simulink model "pv_dq_sim"  (R2014b)
settings: Solver=ode45  SolverMode=SingleTasking  StartTime=0.0  StopTime=2  MaxStep=0.0002  RelTol=0.0001
values from neighbouring files (symbols this model uses):
  C = full(C)    [ex3busPV.m]    (also in ex_get_started_here.m = 5e-07; pv_dq.m = 4.01652892562e-06)
  Kci = Kcp^2/(2*Linv)    [exSyncGenPVinv.m]    (also in pv_dq.m = 3.11562907794)
  Kcp = 10*4*pi*Linv    [exSyncGenPVinv.m]    (also in pv_dq.m = 0.0495867768595)
  Kpi = 0.1*Kpp^2/(Ebus/Vinv_rt)    [exSyncGenPVinv.m]    (also in pv_dq.m = 251.934662919)
  Kpp = 200*(Ebus/Vinv_rt)    [exSyncGenPVinv.m]    (also in pv_dq.m = 12.596733146)
  L = 0.5    [ex2busStability.m]    (also in ex_get_started_here.m = 0.05; pv_dq.m = 0.000394599032459)
  Pdc_op = 0.6*Pinv_rt    [exSyncGenPVinv.m]    (also in pv_dq.m = 1600000)
  Qstar = 0    [exSyncGenPVinv.m]    (also in pv_dq.m)
  ramp_duration = 1    [pv_dq.m]
  ramp_size = -0.1    [pv_dq.m]
  ramp_starts_at = 0.2    [pv_dq.m]
  Vdcset = (2^0.5)*Vinv_rt/duty_max    [exSyncGenPVinv.m]    (also in pv_dq.m = 19958.8053116)
  Vg = 22e3 / 3^0.5    (= 12701.7059222)    [pv_dq.m]
  Vinv_rt = mpc.bus(ssgen(synrp),VM).*baseV(ssgen(synrp))    [exSyncGenPVinv.m]    (also in pv_dq.m = 12701.7059222)
  ws = 2*pi*50    (= 314.159265359)    [ex14busSGandPV.m]    (also in ex2busStability.m; ex3busPV.m; ex7busLongLine.m; ex9busSG.m)
undefined symbols (not defined in the file or in its folder): magnitude
libraries: simulink x1
settings Model: Creator=COPEC  LastModifiedBy=Juri
settings OptimizationCC: BlockReduction=off  BooleanDataType=off
settings DebuggingCC: SaveWithParameterizedLinksMsg=none  UnderspecifiedInitializationDetection=Classic  MergeDetectMultiDrivingBlocksExec=none  SignalResolutionControl=TryResolveAllWithWarning  SolverPrmCheckMsg=none  FrameProcessingCompatibilityMsg=error
settings HardwareCC: TargetUnknown=on

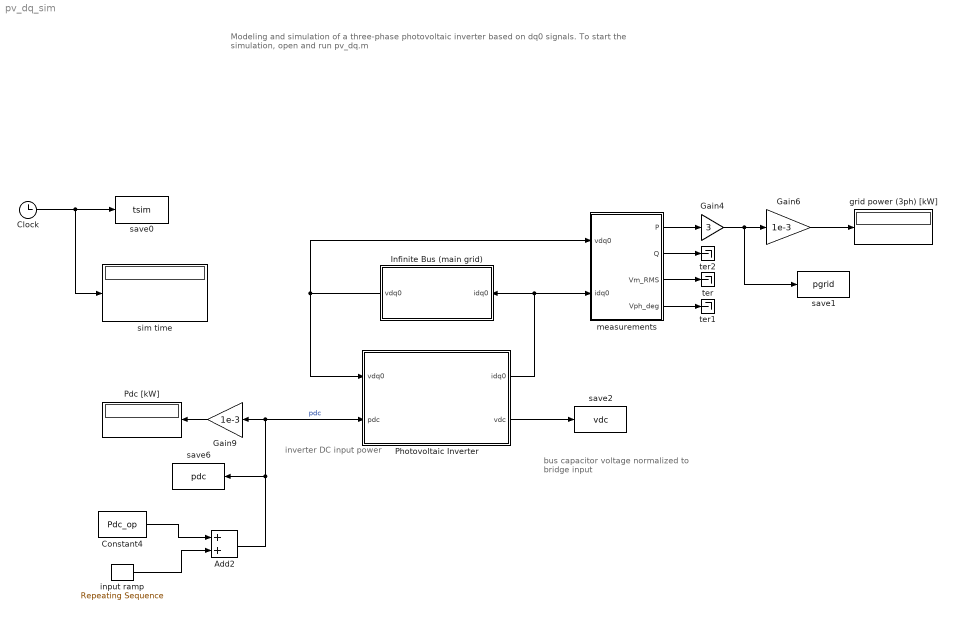
== system pv_dq_sim ==
  note: inverter DC input power
  note: bus capacitor voltage normalized to bridge input
  note: Modeling and simulation of a three-phase
      | photovoltaic inverter based on dq0 signals.
      |
      | To start the simulation, open and run pv_dq.m
  Add2 : Sum
  Clock : Clock
  Constant4 : Constant  Value=Pdc_op
  Gain4 : Gain  Gain=3
  Gain6 : Gain  Gain=1e-3
  Gain9 : Gain  Gain=1e-3
  Infinite Bus (main grid) : Subsystem
  Pdc [kW] : Display
  Photovoltaic Inverter : Subsystem
  grid power (3ph) [kW] : Display
  input ramp : simulink/Sources/Repeating Sequence  rep_seq_t=[0 ramp_starts_at (ramp_starts_at+ramp_duration) 1e6]  rep_seq_y=[0 0 Pdc_op*ramp_size Pdc_op*ramp_size]
  measurements : Subsystem
  save0 : ToWorkspace  VariableName=tsim  SampleTime=-1
  save1 : ToWorkspace  VariableName=pgrid  SampleTime=-1
  save2 : ToWorkspace  VariableName=vdc  SampleTime=-1
  save6 : ToWorkspace  VariableName=pdc  SampleTime=-1
  sim time : Display
  ter : Terminator
  ter1 : Terminator
  ter2 : Terminator
  wires:
  Clock/1 -> sim time/1, save0/1
  Gain6/1 -> grid power (3ph) [kW]/1
  input ramp/1 -> Add2/2
  Gain9/1 -> Pdc [kW]/1
  Constant4/1 -> Add2/1
  Add2/1 -> Photovoltaic Inverter/2(pdc), Gain9/1, save6/1  "pdc"
  Infinite Bus (main grid)/1(vdq0) -> measurements/1(vdq0), Photovoltaic Inverter/1(vdq0)
  Photovoltaic Inverter/1(idq0) -> Infinite Bus (main grid)/1(idq0), measurements/2(idq0)
  measurements/3(Vm_RMS) -> ter/1
  measurements/4(Vph_deg) -> ter1/1
  measurements/2(Q) -> ter2/1
  measurements/1(P) -> Gain4/1
  Gain4/1 -> Gain6/1, save1/1
  Photovoltaic Inverter/2(vdc) -> save2/1

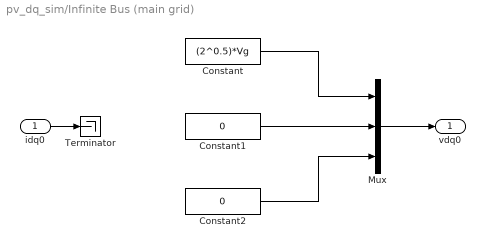
== system pv_dq_sim/Infinite Bus (main grid) ==
  idq0 : Inport
  Constant : Constant  Value=(2^0.5)*Vg
  Constant1 : Constant  Value=0
  Constant2 : Constant  Value=0
  Mux : Mux  Inputs=3
  Terminator : Terminator
  vdq0 : Outport
  wires:
  Mux/1 -> vdq0/1
  Constant/1 -> Mux/1
  Constant1/1 -> Mux/2
  Constant2/1 -> Mux/3
  idq0/1 -> Terminator/1

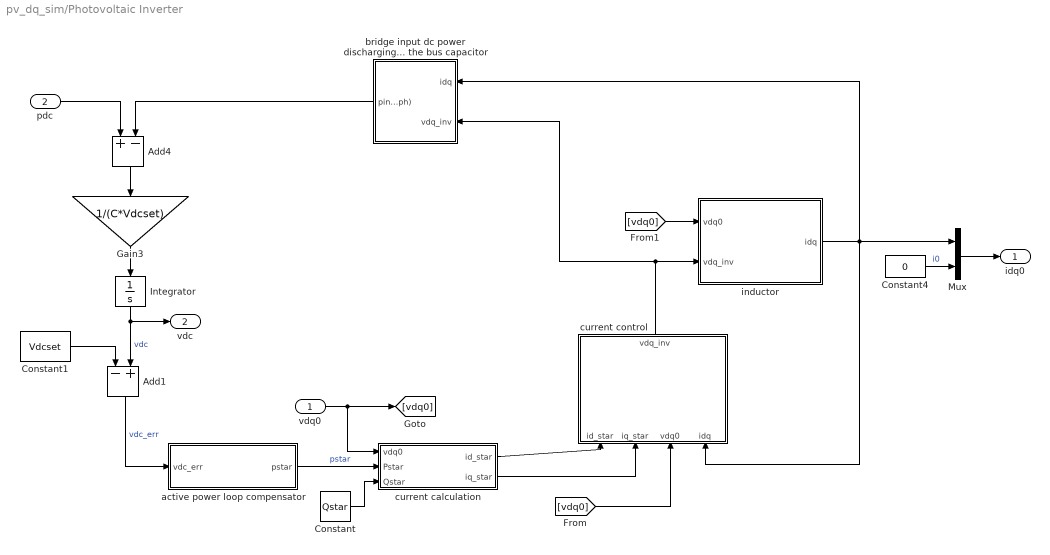
== system pv_dq_sim/Photovoltaic Inverter ==
  vdq0 : Inport
  pdc : Inport  Port=2
  Add1 : Sum  Inputs=-+
  Add4 : Sum  Inputs=+-
  Constant : Constant  Value=Qstar
  Constant1 : Constant  Value=Vdcset
  Constant4 : Constant  Value=0
  Gain3 : Gain  Gain=1/(C*Vdcset)
  Integrator : Integrator  InitialCondition=Vdcset
  Mux : Mux  Inputs=2
  active power loop compensator : Subsystem
  bridge input dc power discharging the bus capacitor : Subsystem
  current control : Subsystem
  current calculation : Subsystem
  inductor : Subsystem
  idq0 : Outport
  vdc : Outport  Port=2
  wires:
  Integrator/1 -> Add1/2, vdc/1  "vdc"
  Constant/1 -> current calculation/3(Qstar)
  Add4/1 -> Gain3/1
  Constant1/1 -> Add1/1
  active power loop compensator/1(pstar) -> current calculation/2(Pstar)  "pstar"
  Gain3/1 -> Integrator/1
  current calculation/2(iq_star) -> current control/2(iq_star)
  current calculation/1(id_star) -> current control/1(id_star)
  Add1/1 -> active power loop compensator/1(vdc_err)  "vdc_err"
  pdc/1 -> Add4/1
  vdq0/1 -> current calculation/1(vdq0), [vdq0]
  [vdq0] -> current control/3(vdq0)
  [vdq0] -> inductor/1(vdq0)
  current control/1(vdq_inv) -> bridge input dc power discharging the bus capacitor/2(vdq_inv), inductor/2(vdq_inv)
  bridge input dc power discharging the bus capacitor/1(pinv (3ph)) -> Add4/2
  Mux/1 -> idq0/1
  inductor/1(idq) -> bridge input dc power discharging the bus capacitor/1(idq), Mux/1, current control/4(idq)
  Constant4/1 -> Mux/2  "i0"

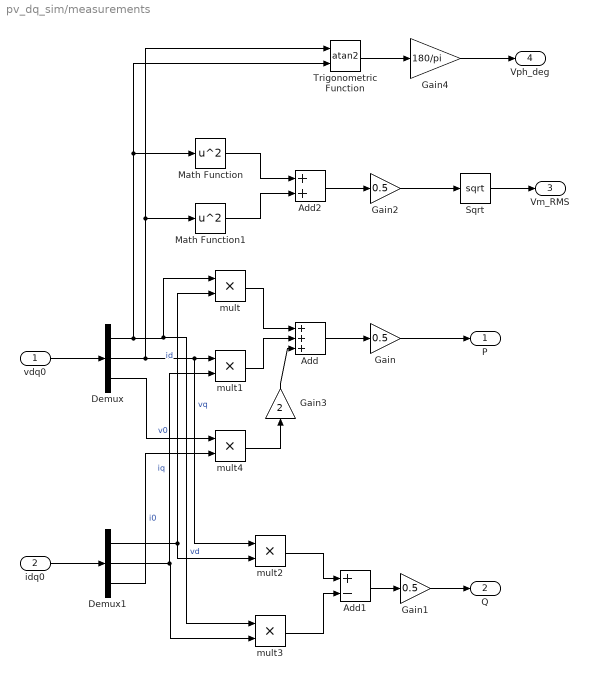
== system pv_dq_sim/measurements ==
  vdq0 : Inport
  idq0 : Inport  Port=2
  Add : Sum  Inputs=+++
  Add1 : Sum  Inputs=+-
  Add2 : Sum
  Demux : Demux  Outputs=3
  Demux1 : Demux  Outputs=3
  Gain : Gain  Gain=0.5
  Gain1 : Gain  Gain=0.5
  Gain2 : Gain  Gain=0.5
  Gain3 : Gain  Gain=2
  Gain4 : Gain  Gain=180/pi
  Math Function : Math  Operator=square  SaturateOnIntegerOverflow=on
  Math Function1 : Math  Operator=square  SaturateOnIntegerOverflow=on
  Sqrt : Sqrt  SaturateOnIntegerOverflow=on
  Trigonometric Function : Trigonometry  Operator=atan2
  mult{,1..4} (5 alike) : Product  Inputs=**
  P : Outport
  Q : Outport  Port=2
  Vm_RMS : Outport  Port=3
  Vph_deg : Outport  Port=4
  wires:
  idq0/1 -> Demux1/1
  vdq0/1 -> Demux/1
  Demux/1 -> Math Function/1, Trigonometric Function/2, mult3/1, mult/1  "vd"
  Demux/2 -> Trigonometric Function/1, Math Function1/1, mult2/1, mult1/1  "vq"
  Demux1/1 -> mult/2, mult2/2  "id"
  Demux1/2 -> mult3/2, mult1/2  "iq"
  Demux/3 -> mult4/1  "v0"
  Demux1/3 -> mult4/2  "i0"
  mult/1 -> Add/1
  mult1/1 -> Add/2
  Add/1 -> Gain/1
  mult2/1 -> Add1/1
  mult3/1 -> Add1/2
  Add1/1 -> Gain1/1
  Sqrt/1 -> Vm_RMS/1
  Math Function/1 -> Add2/1
  Math Function1/1 -> Add2/2
  Add2/1 -> Gain2/1
  Gain2/1 -> Sqrt/1
  Gain/1 -> P/1
  Gain1/1 -> Q/1
  mult4/1 -> Gain3/1
  Gain3/1 -> Add/3
  Trigonometric Function/1 -> Gain4/1
  Gain4/1 -> Vph_deg/1

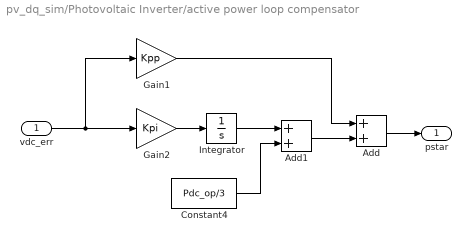
== system pv_dq_sim/Photovoltaic Inverter/active power loop compensator ==
  vdc_err : Inport
  Add : Sum
  Add1 : Sum
  Constant4 : Constant  Value=Pdc_op/3
  Gain1 : Gain  Gain=Kpp
  Gain2 : Gain  Gain=Kpi
  Integrator : Integrator
  pstar : Outport
  wires:
  vdc_err/1 -> Gain2/1, Gain1/1
  Add1/1 -> Add/2
  Gain1/1 -> Add/1
  Gain2/1 -> Integrator/1
  Integrator/1 -> Add1/1
  Constant4/1 -> Add1/2
  Add/1 -> pstar/1

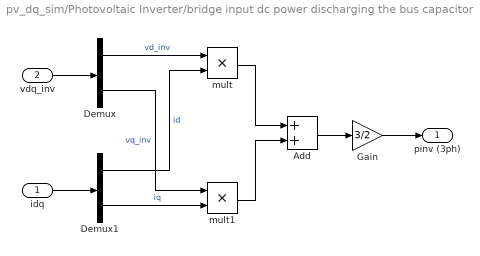
== system pv_dq_sim/Photovoltaic Inverter/bridge input dc power discharging the bus capacitor ==
  idq : Inport
  vdq_inv : Inport  Port=2
  Add : Sum
  Demux : Demux  Outputs=2
  Demux1 : Demux  Outputs=2
  Gain : Gain  Gain=3/2
  mult : Product  Inputs=**
  mult1 : Product  Inputs=**
  pinv (3ph) : Outport
  wires:
  idq/1 -> Demux1/1
  vdq_inv/1 -> Demux/1
  Demux/1 -> mult/1  "vd_inv"
  Demux/2 -> mult1/1  "vq_inv"
  Demux1/1 -> mult/2  "id"
  Demux1/2 -> mult1/2  "iq"
  mult/1 -> Add/1
  mult1/1 -> Add/2
  Add/1 -> Gain/1
  Gain/1 -> pinv (3ph)/1

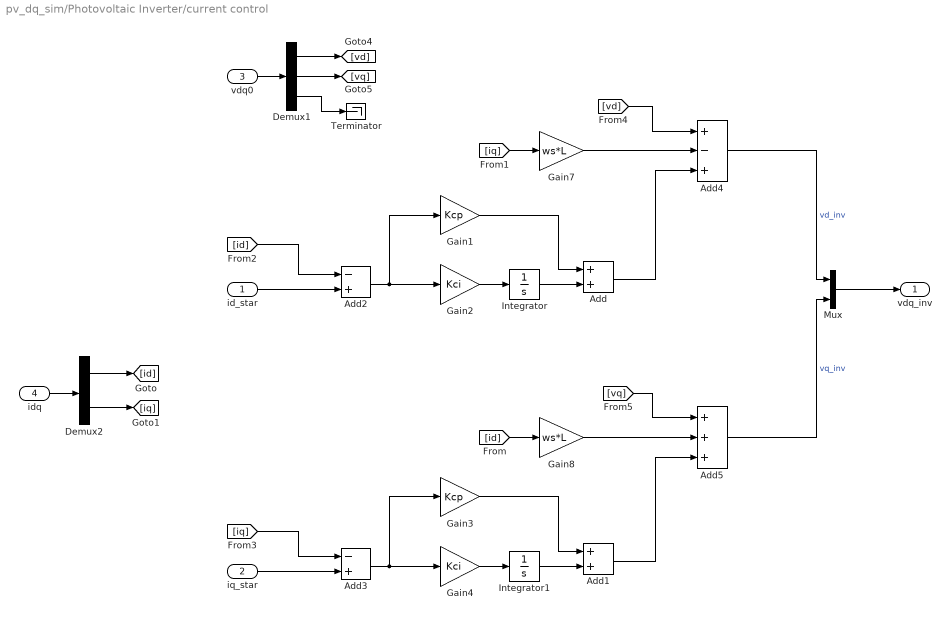
== system pv_dq_sim/Photovoltaic Inverter/current control ==
  id_star : Inport
  iq_star : Inport  Port=2
  vdq0 : Inport  Port=3
  idq : Inport  Port=4
  Add : Sum
  Add1 : Sum
  Add2 : Sum  Inputs=-+
  Add3 : Sum  Inputs=-+
  Add4 : Sum  Inputs=+-+
  Add5 : Sum  Inputs=+++
  Demux1 : Demux  Outputs=3
  Demux2 : Demux  Outputs=2
  Gain1 : Gain  Gain=Kcp
  Gain2 : Gain  Gain=Kci
  Gain3 : Gain  Gain=Kcp
  Gain4 : Gain  Gain=Kci
  Gain7 : Gain  Gain=ws*L
  Gain8 : Gain  Gain=ws*L
  Integrator : Integrator
  Integrator1 : Integrator
  Mux : Mux  Inputs=2
  Terminator : Terminator
  vdq_inv : Outport
  wires:
  Add2/1 -> Gain2/1, Gain1/1
  Integrator/1 -> Add/2
  Add/1 -> Add4/3
  Gain1/1 -> Add/1
  Gain2/1 -> Integrator/1
  Add3/1 -> Gain4/1, Gain3/1
  Integrator1/1 -> Add1/2
  Add1/1 -> Add5/3
  Gain3/1 -> Add1/1
  Gain4/1 -> Integrator1/1
  Add4/1 -> Mux/1  "vd_inv"
  Add5/1 -> Mux/2  "vq_inv"
  id_star/1 -> Add2/2
  iq_star/1 -> Add3/2
  [vd] -> Add4/1
  [vq] -> Add5/1
  Gain7/1 -> Add4/2
  [iq] -> Gain7/1
  Gain8/1 -> Add5/2
  [id] -> Gain8/1
  Mux/1 -> vdq_inv/1
  Demux1/3 -> Terminator/1
  Demux1/2 -> [vq]
  Demux1/1 -> [vd]
  vdq0/1 -> Demux1/1
  Demux2/2 -> [iq]
  Demux2/1 -> [id]
  idq/1 -> Demux2/1
  [id] -> Add2/1
  [iq] -> Add3/1

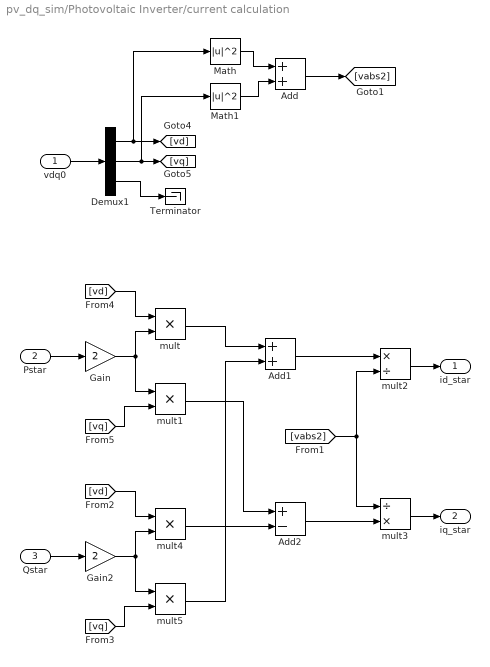
== system pv_dq_sim/Photovoltaic Inverter/current calculation ==
  vdq0 : Inport
  Pstar : Inport  Port=2
  Qstar : Inport  Port=3
  Add : Sum
  Add1 : Sum
  Add2 : Sum  Inputs=+-
  Demux1 : Demux  Outputs=3
  Gain : Gain  Gain=2
  Gain2 : Gain  Gain=2
  Math : Math  Operator=magnitude^2  SaturateOnIntegerOverflow=on
  Math1 : Math  Operator=magnitude^2  SaturateOnIntegerOverflow=on
  Terminator : Terminator
  mult{,1,4..5} (4 alike) : Product  Inputs=**
  mult2 : Product  Inputs=*/
  mult3 : Product  Inputs=/*
  id_star : Outport
  iq_star : Outport  Port=2
  wires:
  Demux1/3 -> Terminator/1
  Demux1/2 -> Math1/1, [vq]
  Demux1/1 -> Math/1, [vd]
  vdq0/1 -> Demux1/1
  Math/1 -> Add/1
  Math1/1 -> Add/2
  Add/1 -> [vabs2]
  Pstar/1 -> Gain/1
  Gain/1 -> mult1/1, mult/2
  [vd] -> mult/1
  [vq] -> mult1/2
  Qstar/1 -> Gain2/1
  Gain2/1 -> mult5/1, mult4/2
  [vd] -> mult4/1
  [vq] -> mult5/2
  mult2/1 -> id_star/1
  [vabs2] -> mult3/1, mult2/2
  mult3/1 -> iq_star/1
  Add1/1 -> mult2/1
  mult/1 -> Add1/1
  mult5/1 -> Add1/2
  mult4/1 -> Add2/2
  mult1/1 -> Add2/1
  Add2/1 -> mult3/2

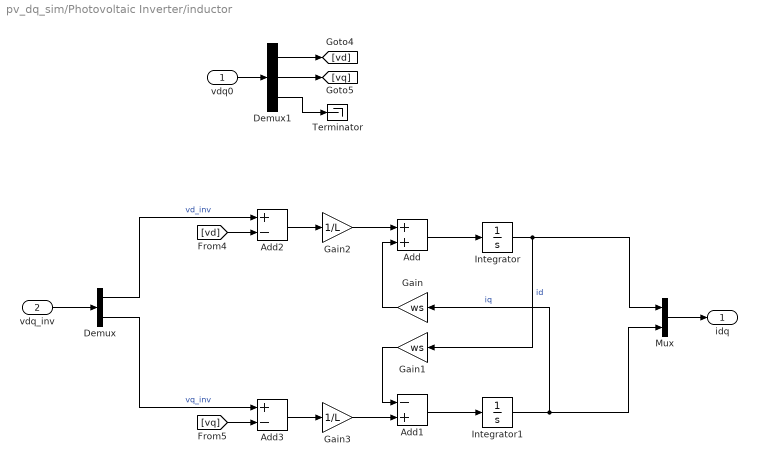
== system pv_dq_sim/Photovoltaic Inverter/inductor ==
  vdq0 : Inport
  vdq_inv : Inport  Port=2
  Add : Sum
  Add1 : Sum  Inputs=-+
  Add2 : Sum  Inputs=+-
  Add3 : Sum  Inputs=+-
  Demux : Demux  Outputs=2
  Demux1 : Demux  Outputs=3
  Gain : Gain  Gain=ws
  Gain1 : Gain  Gain=ws
  Gain2 : Gain  Gain=1/L
  Gain3 : Gain  Gain=1/L
  Integrator : Integrator  InitialCondition=(2^0.5)*(Pdc_op/3)/Vinv_rt
  Integrator1 : Integrator
  Mux : Mux  Inputs=2
  Terminator : Terminator
  idq : Outport
  wires:
  Integrator/1 -> Gain1/1, Mux/1  "id"
  Integrator1/1 -> Mux/2, Gain/1  "iq"
  Add/1 -> Integrator/1
  Add1/1 -> Integrator1/1
  Gain/1 -> Add/2
  Gain1/1 -> Add1/1
  Gain2/1 -> Add/1
  Gain3/1 -> Add1/2
  Demux/1 -> Add2/1  "vd_inv"
  Add2/1 -> Gain2/1
  Add3/1 -> Gain3/1
  Demux/2 -> Add3/1  "vq_inv"
  [vd] -> Add2/2
  [vq] -> Add3/2
  vdq_inv/1 -> Demux/1
  vdq0/1 -> Demux1/1
  Demux1/1 -> [vd]
  Demux1/3 -> Terminator/1
  Demux1/2 -> [vq]
  Mux/1 -> idq/1
